simulink model "CDPR_bloques_lazo_cerrado_3D_parametric_R2020a"  (R2020a)
settings: Solver=ode15s  StartTime=0.0  StopTime=10  MaxStep=0.001  RelTol=1e-30
InitFcn:
  | % The global parameters for simulink are defined by running this script
  | % - Back emf constant           [Kb] (V/rad/sec)
  | % - Motor torque constant       [Kt] (N.m/A)
  | % - Mechanical inertia          [Jm] (kg.m^2)
  | % - Friction coeficient         [Bm] (N.m.s)
  | % - Armature resistance         [Ra] (Ohm)
  | % - Armature inductance         [La] (H)
  | 
  | Kb = 1.25;
  | Kt = 0.516;
  | Jm = 0.0221;
  | Bm = 0.002953;
  | Ra = 2.581;
  | La = 0.0281;
  | r = 5;
  | M = 5;
  | 
  | % Polos deseados
  | Pdc_ee = [-20 -20];         % Polos del controlador de end effector de CD
  | Pdc_motor = [-4 -4];        % Polos del controlador de motor de CD
  | Pdo_motor = [-80 -80];    % Polos del observador de motor de CD
libraries: simulink x5
(part 2 of 2)

== matlab function CDPR_bloques_lazo_cerrado_3D_parametric_R2020a/Planta End Effector/MATLAB Function ==
  data: U input; dX output; X input; p_acc output; Jt input; p_vel output; M parameter
function [dX, p_acc, p_vel]  = PlantaEndEffector(U, X, Jt, M)
%MATRICES
Fext=[0;0;-9.81*M];
ZeroI33 = 0 * eye(3);
a11 = ZeroI33;
a12 = ZeroI33;
a21 = eye(3);
a22 = ZeroI33;
b11 = zeros(3,4);
b21 = (-1/M) * Jt;
c11 = eye(3);
c12 = ZeroI33;
d12 = 1/M*Fext;

f = [0;0;0; d12];

A = [a11 a21; a12 a22];
B = [b11; b21];
C = [c11 c12];
 
dX = A*X + B*U + f ;
p_vel = dX(1:3);
p_acc = dX(4:6);
end

== matlab function CDPR_bloques_lazo_cerrado_3D_parametric_R2020a/Controladores y observadores Motores DC [4] /Controlador y Observador Motor CD2/MATLAB Function2 ==
  data: U input; X input; Y_err input; dX_hat output; Kb parameter; Kt parameter; Jm parameter; Bm parameter; Ra parameter; La parameter; Pdo_motor parameter
function dX_hat = Observador(U, X, Y_err, Kb, Kt, Jm, Bm, Ra, La, Pdo_motor)
a11 = -Ra/La;
a12 = -Kb/La;
a21 =  Kt/Jm;
a22 = -Bm/Jm;
b11 = 1/La;
b22 = 0;
 
A = [a11 a12; a21 a22]; 
B = [b11; b22];
C = [0 1];

Mo1 = [C ;
      C*A];
Ho = (A-Pdo_motor(1)*eye(2))*(A-Pdo_motor(2)*eye(2));
L = -Ho * (Mo1)^(-1) * [0 1].';
%Espacio de estados
dX_hat = A*X + B*U - L*Y_err;
end

== matlab function CDPR_bloques_lazo_cerrado_3D_parametric_R2020a/Controladores y observadores Motores DC [4] /Controlador y Observador Motor CD1/MATLAB Function2 ==
  data: U input; X input; Y_err input; dX_hat output; Kb parameter; Kt parameter; Jm parameter; Bm parameter; Ra parameter; La parameter; Pdo_motor parameter
function dX_hat = Observador(U, X, Y_err, Kb, Kt, Jm, Bm, Ra, La, Pdo_motor)
a11 = -Ra/La;
a12 = -Kb/La;
a21 =  Kt/Jm;
a22 = -Bm/Jm;
b11 = 1/La;
b22 = 0;
 
A = [a11 a12; a21 a22]; 
B = [b11; b22];
C = [0 1];

Mo1 = [C ;
      C*A];
Ho = (A-Pdo_motor(1)*eye(2))*(A-Pdo_motor(2)*eye(2));
L = -Ho * (Mo1)^(-1) * [0 1].';
%Espacio de estados
dX_hat = A*X + B*U - L*Y_err;
end

== matlab function CDPR_bloques_lazo_cerrado_3D_parametric_R2020a/Sistema de motores y carretes [4]/Sistema de motor2/Planta Motor ==
  data: U input; w_dot input; dX output; X input; Kb parameter; Kt parameter; Jm parameter; Bm parameter; Ra parameter; La parameter
function dX  = MotorCD(U, w_dot, X, Kb, Kt, Jm, Bm, Ra, La)
a11 = -Ra/La;
a12 = -Kb/La;
a21 =  Kt/Jm;
a22 = -Bm/Jm;
b11 = 1/La;
b22 = 0;
f11 = 0;
f22 = -1/Jm;
 
A = [a11 a12; a21 a22]; 
B = [b11; b22];

F = [f11; f22];
TL = -Kt * X(1) + Jm * w_dot + Bm * X(2) ;
 
dX = A*X + B*U + F*TL;
end

== matlab function CDPR_bloques_lazo_cerrado_3D_parametric_R2020a/Controlador End Effector/MATLAB Function7 ==
  settings: updateMethod=CONTINUOUS
  data: Yref input; dYref input; ddYref input; Jt input; X input; U output; Err output; Xref output; M parameter; Pdc_ee parameter
function [U, Err, Xref]  = Controlador(Yref, dYref, ddYref, Jt, X, M, Pdc_ee)
% Ubicación de los polos para que el error converja a cero
k1 = Pdc_ee(1);    % Pd bloque 1
k2 = Pdc_ee(2);    % Pd bloque 2
b2 = (-1/M) * Jt;  % valor del B(2);
P = [ 0; 0; -9.81];

% Expresion de los estados; 
x1 = X(1:3);
x2 = X(4:6);

% Ecuaciones de bloques, derivadas de los estados. 
dx1 = x2; 
%dx2 = b2*u + fext;

% Ecuaciones del bloque 1
e1 = Yref - x1;                                                     % 5.4
de1 =  k1 * e1;                                                     % 5.5a
x2ref = dYref  - de1;                                               % 5.6b

% Dinamica de x3ref
dx2ref = ddYref - k1*dYref + k1*dx1;                                % 5.8

% Ecuaciones del bloque 2
e2 = x2ref - x2;                                                    % 5.9
de2 = k2*e2;                                                        % 5.10a

% Salidas del bloque, Ley de control, error y estados de referencia.
U = (pinv(b2))*(dx2ref - de2 - P);                         % 5.16b

Err = [e1; e2];
Xref = x2ref;
end
